simulink model "doc_mlse_dynamic_coeffs"  (R2014a)
settings: Solver=VariableStepDiscrete  StartTime=0.0  StopTime=10.0  RelTol=1e-3
undefined symbols (not defined in the file or in its folder): j
libraries: commchan3 x2, commdigbbndpm3 x2, commrandsrc2 x1, commsink2 x1, commeq2 x1
settings Model: ExtModeAutoUpdateStatusClock=off  Creator=The MathWorks Inc.
settings DataIOCC: SignalLoggingSaveFormat=ModelDataLogs
settings OptimizationCC: ExpressionDepthLimit=2147483647  InitFltsAndDblsToZero=on
settings DebuggingCC: SaveWithParameterizedLinksMsg=none  UnderspecifiedInitializationDetection=Classic  SignalResolutionControl=TryResolveAllWithWarning  FcnCallInpInsideContextMsg=UseLocalSettings  StateNameClashWarn=warning  StrictBusMsg=Warning
settings GRTTargetCC: TargetFcnLib=ansi_tfl_tmw.mat  CombineOutputUpdateFcns=off  GRTInterface=on

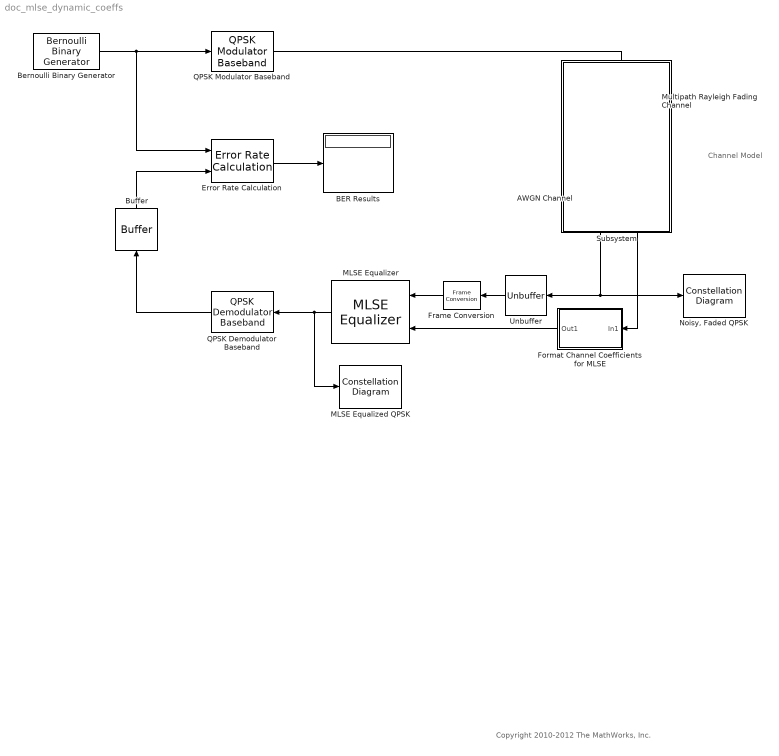
== system doc_mlse_dynamic_coeffs ==
  note: Channel
      | Model
  note: Copyright 2010-2012 The MathWorks, Inc.
  AWGN Channel : commchan3/AWGN Channel  InputProcessing=Columns as channels (frame based)  seed=67  noiseMode="Signal to noise ratio  (SNR)"  EbNodB=10  EsNodB=10  SNRdB=10  bitsPerSym=1  Ps=1  Tsym=1  variance=0.3
  BER Results : Display
  Bernoulli Binary Generator : commrandsrc2/Bernoulli Binary Generator  P=0.5  seed=9973  Ts=5e-6  frameBased=on  sampPerFrame=100  orient=off  outDataType=double
  Buffer : Buffer  N=100  TreatMby1Signals=One channel
  Error Rate Calculation : commsink2/Error Rate Calculation  N=120  st_delay=400  cp_mode=Entire frame  subframe=[]  PMode=Port  WsName=ErrorVec  RsMode2=off  stop=on  numErr=500  maxBits=1e6
  Format Channel Coefficients for MLSE : Subsystem
  Frame Conversion : FrameConversion
  MLSE Equalized QPSK : ConstellationDiagram  Tag=ScatterPlot
  MLSE Equalizer : commeq2/MLSE Equalizer  specchan=Input port  chancoeff=fir1(5, 0.5)  constpts=[1+j -1+j 1-j -1-j]/sqrt(2)  tbdepth=10  opmode=Continuous with reset option  enpreamble=off  preamble=[ones(1,8)]  enpostamble=off  postamble=[0 2 3 1]  numsamp=1  reset=off
  Multipath Rayleigh Fading Channel : commchan3/Multipath Rayleigh Fading Channel  maxDopplerShift=30  spectrumType=Jakes  sigmaGaussian=1/sqrt(2)  coeffRounded=[1 -1.72 0.785]  freqMinMaxRJakes=[0 1]  freqMinMaxAJakes=[0 1]  sigmaGaussian1=1/sqrt(2)  sigmaGaussian2=1/sqrt(2)  centerFreqGaussian1=0.0  centerFreqGaussian2=0.0  gainGaussian1=0.5  gainGaussian2=0.5  coeffBell=9  dopplerSpectrum=doppler.jakes  pathDelays=[0 5e-4/50]  avgPathGaindB=[0 -10]  normalizePathGains=on  seed=73  enableProbe=1  openVisAtStart=on  outPathGains=on  outDelay=off
  "Noisy, Faded QPSK" : ConstellationDiagram  Tag=ScatterPlot
  QPSK Demodulator Baseband : commdigbbndpm3/QPSK Demodulator Baseband  Ph=pi/4  Dec=Gray  OutType=Bit  DecType=Hard decision  VarSource=Dialog  Variance=1  outDtype1=double  outDtype2=double  derotateFactorWordLen=16
  QPSK Modulator Baseband : commdigbbndpm3/QPSK Modulator Baseband  InType=Bit  Enc=Gray  Ph=pi/4  outDtype=double  outWordLen=16  outUDDataType=sfix(16)  outFracLenMode=Best precision  outFracLen=15
  Subsystem : Subsystem
      mask Display: disp('')
  Unbuffer : Unbuffer  SampleBasedProcessing=Same as frame based
  wires:
  Error Rate Calculation/1 -> BER Results/1
  Bernoulli Binary Generator/1 -> QPSK Modulator Baseband/1, Error Rate Calculation/1
  MLSE Equalizer/1 -> QPSK Demodulator Baseband/1, MLSE Equalized QPSK/1
  AWGN Channel/1 -> "Noisy, Faded QPSK"/1, Unbuffer/1
  QPSK Demodulator Baseband/1 -> Buffer/1
  Format Channel Coefficients for MLSE/1(Out1) -> MLSE Equalizer/2
  Frame Conversion/1 -> MLSE Equalizer/1
  Unbuffer/1 -> Frame Conversion/1
  QPSK Modulator Baseband/1 -> Multipath Rayleigh Fading Channel/1
  Multipath Rayleigh Fading Channel/1 -> AWGN Channel/1
  Multipath Rayleigh Fading Channel/2 -> Format Channel Coefficients for MLSE/1(In1)
  Buffer/1 -> Error Rate Calculation/2

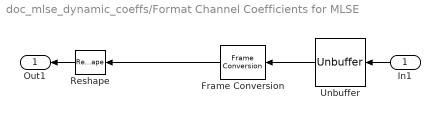
== system doc_mlse_dynamic_coeffs/Format Channel Coefficients for MLSE ==
  In1 : Inport
  Frame Conversion : FrameConversion
  Reshape : Reshape  OutputDimensionality=Column vector (2-D)
  Unbuffer : Unbuffer  SampleBasedProcessing=Same as frame based
  Out1 : Outport
  wires:
  Unbuffer/1 -> Frame Conversion/1
  Reshape/1 -> Out1/1
  In1/1 -> Unbuffer/1
  Frame Conversion/1 -> Reshape/1

== system doc_mlse_dynamic_coeffs/Subsystem ==
